simulink model "hgv_longitudinal_closed_loop"  (R2023b)
settings: Solver=FixedStepDiscrete  StartTime=0.0  StopTime=45  FixedStep=0.02  RelTol=1e-3
settings Model: Creator=luoman  LastModifiedBy=luoman

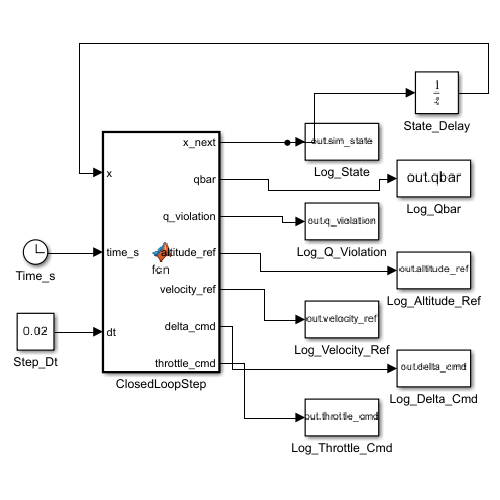
[thumbnail: Simulink's stored preview of the top-level diagram]
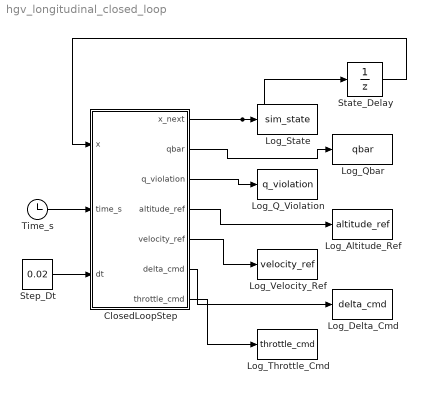
== system hgv_longitudinal_closed_loop ==
  ClosedLoopStep : MATLAB Function  TreatAsAtomicUnit=on
  Log_Altitude_Ref : ToWorkspace  VariableName=altitude_ref  SampleTime=-1
  Log_Delta_Cmd : ToWorkspace  VariableName=delta_cmd  SampleTime=-1
  Log_Q_Violation : ToWorkspace  VariableName=q_violation  SampleTime=-1
  Log_Qbar : ToWorkspace  VariableName=qbar  SampleTime=-1
  Log_State : ToWorkspace  VariableName=sim_state  SampleTime=-1
  Log_Throttle_Cmd : ToWorkspace  VariableName=throttle_cmd  SampleTime=-1
  Log_Velocity_Ref : ToWorkspace  VariableName=velocity_ref  SampleTime=-1
  State_Delay : UnitDelay  InitialCondition=[1750;30000;deg2rad(-0.5);deg2rad(2.0);0;deg2rad(1.5);0;0]  SampleTime=0.02  HasFrameUpgradeWarning=on
  Step_Dt : Constant  Value=0.02
  Time_s : Clock
  wires:
  ClosedLoopStep/7(throttle_cmd) -> Log_Throttle_Cmd/1
  ClosedLoopStep/6(delta_cmd) -> Log_Delta_Cmd/1
  ClosedLoopStep/5(velocity_ref) -> Log_Velocity_Ref/1
  ClosedLoopStep/4(altitude_ref) -> Log_Altitude_Ref/1
  ClosedLoopStep/3(q_violation) -> Log_Q_Violation/1
  ClosedLoopStep/2(qbar) -> Log_Qbar/1
  Step_Dt/1 -> ClosedLoopStep/3(dt)
  Time_s/1 -> ClosedLoopStep/2(time_s)
  State_Delay/1 -> ClosedLoopStep/1(x)
  ClosedLoopStep/1(x_next) -> State_Delay/1, Log_State/1

== matlab function hgv_longitudinal_closed_loop/ClosedLoopStep ==
  data: x input; x_next output; time_s input; dt input; qbar output; q_violation output; altitude_ref output; velocity_ref output; delta_cmd output; throttle_cmd output
function [x_next,qbar,q_violation,altitude_ref,velocity_ref,delta_cmd,throttle_cmd] = fcn(x,time_s,dt)
% Guarded longitudinal closed-loop step for tutorial simulation.
q_limit = 70000.0;
q_warning = 62000.0;
altitude_ref = 30000.0 - 900.0 * min(1.0, time_s / 35.0);
velocity_ref = 1750.0 + 80.0 * min(1.0, time_s / 25.0);
qbar = dyn_pressure(x);
altitude_cmd = altitude_ref;
velocity_cmd = velocity_ref;
if qbar > q_warning
    severity = min(1.0, (qbar - q_warning) / max(1.0, q_limit - q_warning));
    altitude_cmd = altitude_ref + severity * 7000.0;
    velocity_cmd = max(900.0, velocity_ref - severity * 500.0);
end
[delta_cmd, throttle_cmd] = baseline_command(x, altitude_cmd, velocity_cmd);
x_next = rk4_step(x, delta_cmd, throttle_cmd, dt);
q_violation = max(0.0, qbar - q_limit);
end

function [delta_cmd, throttle_cmd] = baseline_command(x, altitude_ref, velocity_ref)
h_gain = 1.5e-4;
gamma_gain = 1.15;
q_gain = 0.55;
v_gain = 7.0e-4;
trim_throttle = 0.62;
alpha_trim = 2.0*pi/180.0;
delta_limit = 18.0*pi/180.0;
gamma_cmd = clamp(h_gain * (altitude_ref - x(2)), -8.0*pi/180.0, 8.0*pi/180.0);
alpha_cmd = alpha_trim + clamp(gamma_gain * (gamma_cmd - x(3)), -5.0*pi/180.0, 5.0*pi/180.0);
theta_cmd = alpha_cmd + x(3);
delta_cmd = -0.9 * (theta_cmd - x(6)) + q_gain * x(5);
delta_cmd = clamp(delta_cmd, -delta_limit, delta_limit);
throttle_cmd = trim_throttle + v_gain * (velocity_ref - x(1));
throttle_cmd = clamp(throttle_cmd, 0.0, 1.0);
end

function x_next = rk4_step(x, delta_cmd, throttle_cmd, dt)
k1 = derivatives(x, delta_cmd, throttle_cmd);
k2 = derivatives(add_state(x, k1, 0.5*dt), delta_cmd, throttle_cmd);
k3 = derivatives(add_state(x, k2, 0.5*dt), delta_cmd, throttle_cmd);
k4 = derivatives(add_state(x, k3, dt), delta_cmd, throttle_cmd);
x_next = x + dt * (k1 + 2*k2 + 2*k3 + k4) / 6.0;
x_next(1) = max(100.0, x_next(1));
x_next(2) = max(0.0, x_next(2));
x_next(4) = clamp(x_next(4), -12.0*pi/180.0, 18.0*pi/180.0);
x_next(7) = clamp(x_next(7), -18.0*pi/180.0, 18.0*pi/180.0);
x_next(8) = clamp(x_next(8), -80.0*pi/180.0, 80.0*pi/180.0);
end

function y = add_state(x, dx, scale)
y = x + scale * dx;
y(7) = clamp(y(7), -25.0*pi/180.0, 25.0*pi/180.0);
y(8) = clamp(y(8), -120.0*pi/180.0, 120.0*pi/180.0);
end

function dx = derivatives(x, delta_cmd, throttle_cmd)
mass = 1200.0;
iy = 8.5e4;
ref_area = 1.2;
ref_chord = 3.0;
gravity = 9.80665;
thrust_max = 55000.0;
cl0 = 0.04;
cl_alpha = 2.2;
cl_delta = 0.25;
cd0 = 0.045;
cd_alpha2 = 0.85;
cm_alpha = -0.42;
cm_q = -5.0;
cm_delta = -0.75;
actuator_wn = 22.0;
actuator_zeta = 0.75;
delta_limit = 18.0*pi/180.0;
delta_rate_limit = 80.0*pi/180.0;
delta_cmd = clamp(delta_cmd, -delta_limit, delta_limit);
throttle_cmd = clamp(throttle_cmd, 0.0, 1.0);
qbar_local = dyn_pressure(x);
velocity = max(100.0, x(1));
alpha = x(4);
delta = x(7);
cl = cl0 + cl_alpha * alpha + cl_delta * delta;
cd = cd0 + cd_alpha2 * alpha * alpha;
cm = cm_alpha * alpha + cm_q * (ref_chord / (2.0 * velocity)) * x(5) + cm_delta * delta;
lift = qbar_local * ref_area * cl;
drag = qbar_local * ref_area * cd;
moment = qbar_local * ref_area * ref_chord * cm;
thrust = thrust_max * throttle_cmd;
delta_accel = actuator_wn * actuator_wn * (delta_cmd - x(7)) - 2.0 * actuator_zeta * actuator_wn * x(8);
if abs(x(8)) >= delta_rate_limit && x(8) * delta_accel > 0.0
    delta_accel = 0.0;
end
v_dot = (thrust * cos(alpha) - drag) / mass - gravity * sin(x(3));
gamma_dot = (thrust * sin(alpha) + lift) / (mass * velocity) - gravity * cos(x(3)) / velocity;
h_dot = x(1) * sin(x(3));
q_dot = moment / iy;
theta_dot = x(5);
alpha_dot = theta_dot - gamma_dot;
dx = zeros(8,1);
dx(1) = v_dot;
dx(2) = h_dot;
dx(3) = gamma_dot;
dx(4) = alpha_dot;
dx(5) = q_dot;
dx(6) = theta_dot;
dx(7) = x(8);
dx(8) = delta_accel;
end

function qbar = dyn_pressure(x)
rho0 = 1.225;
scale_height = 7200.0;
rho = rho0 * exp(-max(0.0, x(2)) / scale_height);
qbar = 0.5 * rho * x(1) * x(1);
end

function y = clamp(value, lower, upper)
y = max(lower, min(upper, value));
end
